simulink model "QPSK_TX_SEC6"  (R2021b)
settings: Solver=ode45  StartTime=0.0  StopTime=2000  RelTol=1e-3  EnableMultiTasking=on
libraries: commfilt2 x2, commrandsrc2 x2, commutil2 x2, simulink x1
settings Model: Creator=my2  LastModifiedBy=82102
settings SolverCC: AlgebraicLoopSolver=TrustRegion
settings DataIOCC: LimitDataPoints=on  SaveFormat=Array  SignalLoggingSaveFormat=ModelDataLogs  ReturnWorkspaceOutputs=off
settings OptimizationCC: LifeSpan=inf
settings DebuggingCC: UnderspecifiedInitializationDetection=Classic  MergeDetectMultiDrivingBlocksExec=none  SolverPrmCheckMsg=warning  MultiTaskDSMMsg=warning  MultiTaskCondExecSysMsg=none  FcnCallInpInsideContextMsg=warning  SFUnexpectedBacktrackingDiag=warning  SFNoUnconditionalDefaultTransitionDiag=warning  SFExecutionAtInitializationDiag=none  SFMachineParentedDataDiag=warning  ArithmeticOperatorsInVariantConditions=warning
settings HardwareCC: ProdBitPerPointer=32  ProdBitPerSizeT=32  ProdBitPerPtrDiffT=32  ProdLargestAtomicFloat=None  ProdIntDivRoundTo=Undefined  ProdEndianess=Unspecified  ProdWordSize=32  ProdHWDeviceType=32-bit Generic
settings ModelReferenceCC: PropagateSignalLabelsOutOfModel=off
settings SFSimCC: SimUseLocalCustomCode=off  CustomCodeUndefinedFunction=UseInterfaceOnly
settings RTWCC: RTWUseLocalCustomCode=off
settings CodeAppCC: StateflowObjectComments=on
settings GRTTargetCC: TargetLangStandard=C89/C90 (ANSI)  CombineOutputUpdateFcns=off  GRTInterface=on
settings ConfigComp: CovMetricSettings=dw  CovSaveCumulativeToWorkspaceVar=on  CovSaveSingleToWorkspaceVar=on  CovExternalEMLEnable=off

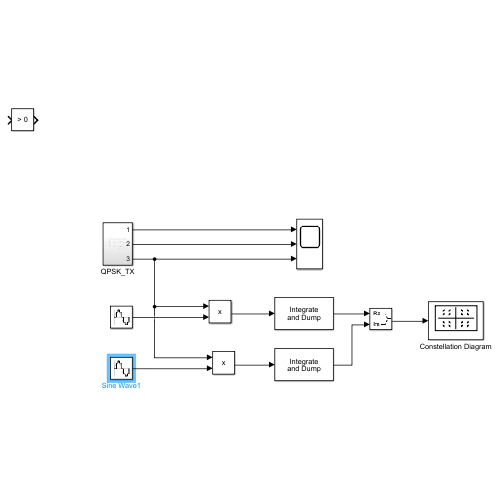
[thumbnail: Simulink's stored preview of the top-level diagram]
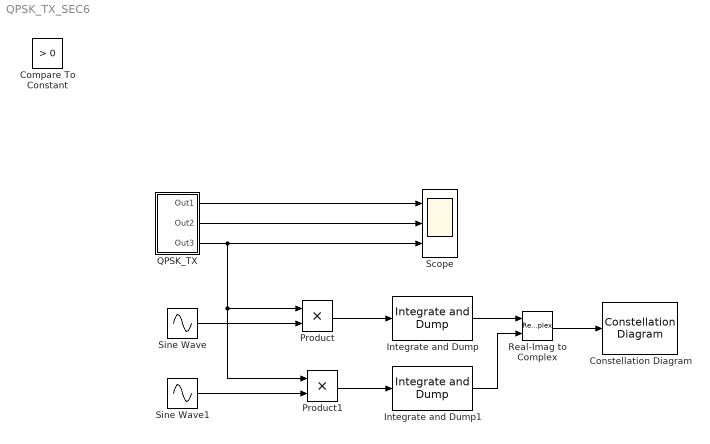
== system QPSK_TX_SEC6 ==
  Compare To Constant : simulink/Logic and Bit Operations/Compare To Constant  relop=>  const=0  OutDataTypeStr=boolean
  Constellation Diagram : ConstellationDiagram  Tag=ScatterPlot
  Integrate and Dump : commfilt2/Integrate and Dump  obssamples=256  offsetsamples=0  nodump=off  roundingMode=Floor  overflowMode=off  outputDataTypeStr=Inherit: Same as accumulator  outputLastDataTypeStr=Inherit: Same as accumulator
  Integrate and Dump1 : commfilt2/Integrate and Dump  obssamples=256  offsetsamples=0  nodump=off  roundingMode=Floor  overflowMode=off  outputDataTypeStr=Inherit: Same as accumulator  outputLastDataTypeStr=Inherit: Same as accumulator
  Product : Product
  Product1 : Product
  QPSK_TX : Subsystem
  Real-Imag to Complex : RealImagToComplex
  Scope : Scope  NumInputPorts=3
  Sine Wave : Sin  Amplitude=sqrt(2)  Frequency=60*pi  Phase=pi/2+pi/3  SampleTime=3.90625e-3
  Sine Wave1 : Sin  Amplitude=sqrt(2)  Frequency=60*pi  Phase=pi/3  SampleTime=3.90625e-3
  wires:
  QPSK_TX/3(Out3) -> Product1/1, Product/1, Scope/3
  Sine Wave/1 -> Product/2
  Product/1 -> Integrate and Dump/1
  Sine Wave1/1 -> Product1/2
  Product1/1 -> Integrate and Dump1/1
  QPSK_TX/1(Out1) -> Scope/1
  QPSK_TX/2(Out2) -> Scope/2
  Integrate and Dump/1 -> Real-Imag to Complex/1
  Integrate and Dump1/1 -> Real-Imag to Complex/2
  Real-Imag to Complex/1 -> Constellation Diagram/1

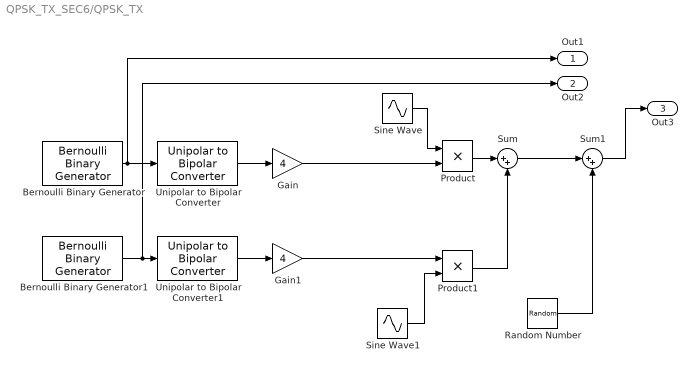
== system QPSK_TX_SEC6/QPSK_TX ==
  Bernoulli Binary Generator : commrandsrc2/Bernoulli Binary Generator  P=0.5  seed=25  Ts=1  frameBased=off  sampPerFrame=1  orient=off  outDataType=boolean
      settings: SourceProductBaseCode=CM
  Bernoulli Binary Generator1 : commrandsrc2/Bernoulli Binary Generator  P=0.5  seed=61  Ts=1  frameBased=off  sampPerFrame=1  orient=off  outDataType=boolean
      settings: SourceProductBaseCode=CM
  Gain : Gain  Gain=4
  Gain1 : Gain  Gain=4
  Product : Product
  Product1 : Product
  Random Number : RandomNumber  Variance=0  Seed=41  SampleTime=1/256  VectorParams1D=off
  Sine Wave : Sin  Amplitude=sqrt(2)  Frequency=60*pi  Phase=pi/2  SampleTime=3.90625e-3
  Sine Wave1 : Sin  Amplitude=sqrt(2)  Frequency=60*pi  SampleTime=3.90625e-3
  Sum : Sum  Inputs=|++
  Sum1 : Sum  Inputs=|++
  Unipolar to Bipolar Converter : commutil2/Unipolar to Bipolar Converter  M=2  polarity=Positive  dataType=Inherit via internal rule
  Unipolar to Bipolar Converter1 : commutil2/Unipolar to Bipolar Converter  M=2  polarity=Positive  dataType=Inherit via internal rule
  Out1 : Outport
  Out2 : Outport  Port=2
  Out3 : Outport  Port=3
  wires:
  Unipolar to Bipolar Converter1/1 -> Gain1/1
  Sine Wave/1 -> Product/1
  Product1/1 -> Sum/2
  Bernoulli Binary Generator/1 -> Out1/1, Unipolar to Bipolar Converter/1
  Gain1/1 -> Product1/1
  Unipolar to Bipolar Converter/1 -> Gain/1
  Sine Wave1/1 -> Product1/2
  Bernoulli Binary Generator1/1 -> Out2/1, Unipolar to Bipolar Converter1/1
  Product/1 -> Sum/1
  Gain/1 -> Product/2
  Random Number/1 -> Sum1/2
  Sum/1 -> Sum1/1
  Sum1/1 -> Out3/1
